simulink library "cdsWD"  (Simulink 6.2)
settings Model: LastModifiedBy=rolf

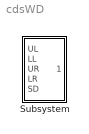
== system cdsWD ==
  Subsystem : Subsystem

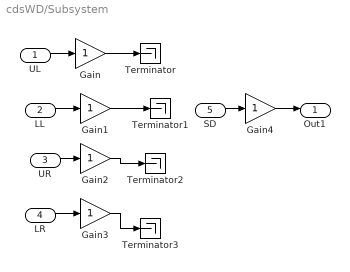
== system cdsWD/Subsystem ==
  UL : Inport  Port=1  LatchInput=off
  LL : Inport  Port=2  LatchInput=off
  UR : Inport  Port=3  LatchInput=off
  LR : Inport  Port=4  LatchInput=off
  SD : Inport  Port=5  LatchInput=off
  Gain{,1..4} (5 alike) : Gain
  Terminator{,1..3} (4 alike) : Terminator
  Out1 : Outport
  wires:
  Gain/1 -> Terminator/1
  Gain3/1 -> Terminator3/1
  Gain2/1 -> Terminator2/1
  Gain1/1 -> Terminator1/1
  UL/1 -> Gain/1
  LL/1 -> Gain1/1
  Gain4/1 -> Out1/1
  SD/1 -> Gain4/1
  UR/1 -> Gain2/1
  LR/1 -> Gain3/1
